simulink subsystem "PvtSubSys_VSM_ALL"  (R2020b)
settings: Solver=VariableStepAuto  StartTime=0.0  StopTime=10.0  RelTol=1e-3
values from neighbouring files (symbols this model uses):
  P_VSM_NOH_Act_Req = 0    [VSM_All.sldd]
  P_VSM_NOH_Swt_Req = 0    [VSM_All.sldd]
undefined symbols (not defined in the file or in its folder): ACC_STATE, HWA_STATE, LCK_STATE, P_VSM_ACCSOS_SW, P_VSM_AESSwtReq, P_VSM_CruiseFunUserInputMappingWays, P_VSM_ELKSwtReq, P_VSM_ESS_VehSwtReq, P_VSM_HWA_DMS_Enable, P_VSM_ICA_HandsOffSwtReq, P_VSM_IntelligentEvaSwtReq, P_VSM_ISLSwtReq, P_VSM_LCKSwtReq, P_VSM_LDWSwtReq, P_VSM_LKASwtReq, P_VSM_LSSSwtReq, P_VSM_PowerTrainConfig, P_VSM_SOSContinueTime, P_VSM_SOSSpdLimit, P_VSM_TSR_Dis_keep_SPL_Table, P_VSM_TSR_Dis_keep_SPLend, P_VSM_TSR_Dis_keep_TS_Table, P_VSM_TSR_Ena_SPLSupp_Table, P_VSM_TSR_Ena_TS_Table, P_VSM_TSR_SLIF_Speed_High, P_VSM_TSR_SLIF_Speed_Low, P_VSM_TSR_SLW_SnvtySwitch, P_VSM_TSR_SLW_Speed_Delta_disable, P_VSM_TSR_SLW_Speed_Delta_enable, P_VSM_TSR_SLW_Speed_High, P_VSM_TSR_SLW_Speed_Low, P_VSM_TSR_SLW_TrafEyeAvtiveDist, P_VSM_TSR_SLW_Warning_Time, P_VSM_TSR_SteerWheelAngle, P_VSM_TSR_SWS_speed_withDir, P_VSM_TSR_SWS_speed_woDir, P_VSM_TSRSwtReq, P_VSM_TSRWarnSwtReq, TJA_STATE, User_LC_ALCswt, User_LC_DrvConfirm, User_LC_DrvLCswt, User_LC_DrvOverride, User_LC_LeTurnNextLineReq, User_LC_RiTurnNextLineReq, User_LC_TurnMostLeLineReq, User_LC_TurnMostRiLineReq, User_LeTurnLmpOn, User_RiTurnLmpOn
libraries: simulink x51
(part 6 of 7)

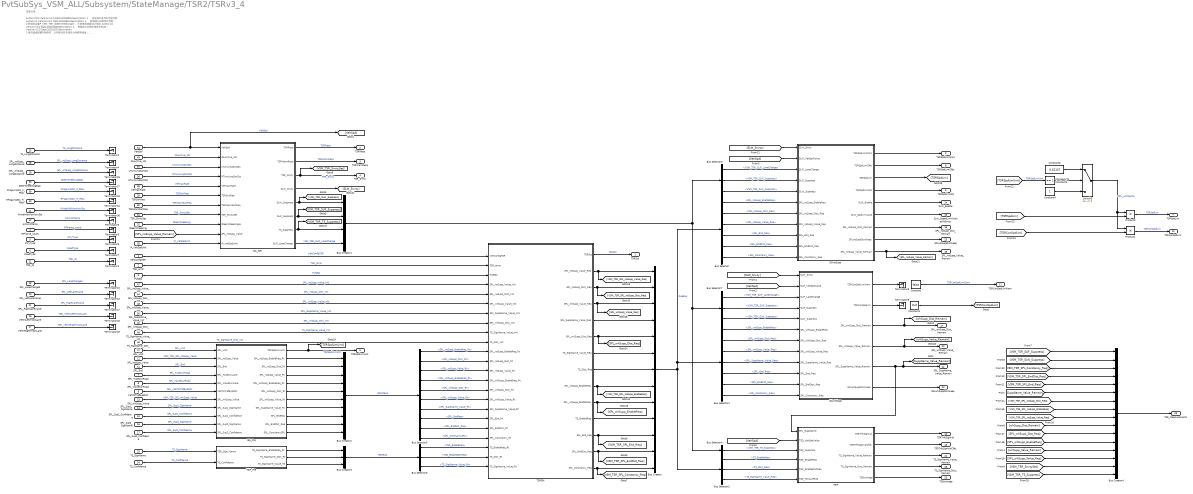
== system PvtSubSys_VSM_ALL/Subsystem/StateManage/TSR2/TSRv3_4 ==
  note: 变更记录
  note: Author:CZN
      | Version:V3.0
      | Data:20200919
      | Description:
      | 1.实现海外版TSR全部功能
      | Author:LC
      | Version:V3.1
      | Data:20200919
      | Description:
      | 1.新增掉头抑制条件判断；
      | 2.新增标定量P_VSM_TSR_SteerWheelAngle；
      | 3.新增观测量CAN输出
      | Author:LC
      | Version:V3.2
      | Data:20201008
      | Description:
      | 1.修复掉头抑制车速条件BUG；
      | Version:V3.3
      | Data:20201102
      | Description:
      | 1.修改超速报警抑制条件，从判断当前车速改为判断限速值；
      | 2.修改TSR_error条件下的状态跳转
      | 3.增加了灵敏度设置限幅；
      | 4.更改SLW_Enable信号来源；
      | 5.修复车速单位为英里时，报警值为公里数值问题；
      | 6.更改限速报警限速策略,改为融合发出信息就显示；
      | Version:V3.4
      | Data:20201103
      | Description:
      | 1、新增三个观测量；
      | 2、新增限速使能触发判断；
      | Version:V3.5
      | Data:20201105
      | Description:
      | 1、按照《交通标志信息功能规范》，新增仪表双位灯输出策略；
      | Version:V3.6
      | Data:20201201
      | Description:
      | 1、条件限速使能改为触发式；
  VehConfigTSR : Inport  OutDataTypeStr=uint8
  TSR_error : Inport  Port=2  OutDataTypeStr=uint8
  FUSSts : Inport  Port=3  OutDataTypeStr=uint8
  RFframe_count : Inport  Port=4  OutDataTypeStr=uint32
  CtryType : Inport  Port=5  OutDataTypeStr=uint8
  RoadType : Inport  Port=6  OutDataTypeStr=uint8
  SPL_TypeCurRoad : Inport  Port=7  OutDataTypeStr=uint8
  SPL_ValueCurRoad : Inport  Port=8  OutDataTypeStr=uint8
  VehToTrafEyeDist : Inport  Port=9  OutDataTypeStr=uint16
  SPL_Unit : Inport  Port=10  OutDataTypeStr=uint8
  SPL_End : Inport  Port=11  OutDataTypeStr=uint8
  SPL_noSupp_Value : Inport  Port=12  OutDataTypeStr=uint8
  SPL_whSupp_Value : Inport  Port=13  OutDataTypeStr=uint8
  SPL_Sup1_SignName : Inport  Port=14  OutDataTypeStr=uint8
  SPL_Sup1_Confidence : Inport  Port=15  OutDataTypeStr=single
  SPL_Sup2_SignName : Inport  Port=16  OutDataTypeStr=uint8
  SPL_Sup2_Confidence : Inport  Port=17  OutDataTypeStr=single
  SPL_noSupp_LongDistance : Inport  Port=18  OutDataTypeStr=uint8
  SPL_whSupp_LongDistance : Inport  Port=19  OutDataTypeStr=uint8
  SPL_LeftLaneValue : Inport  Port=20  OutDataTypeStr=uint8
  SPL_RightLaneValue : Inport  Port=21  OutDataTypeStr=uint8
  TSR_ID : Inport  Port=22  OutDataTypeStr=uint8
  TS_SignName : Inport  Port=23  OutDataTypeStr=uint8
  TS_Confidence : Inport  Port=24  OutDataTypeStr=single
  TS_LongDistance : Inport  Port=25  OutDataTypeStr=uint8
  VehInLeftmostLane : Inport  Port=26  OutDataTypeStr=uint8
  VehInRightmostLane : Inport  Port=27  OutDataTypeStr=uint8
  SPL_LaneChanged : Inport  Port=28  OutDataTypeStr=uint8
  TSRSwtReq : Inport  Port=29  OutDataTypeStr=boolean
  TSRWarnSwtReq : Inport  Port=30  OutDataTypeStr=boolean
  TSR_SnvtySet : Inport  Port=31  OutDataTypeStr=int8
  SteerWheelAng : Inport  Port=32  OutDataTypeStr=single
  SteerWheelAngSign : Inport  Port=33  OutDataTypeStr=boolean
  VehSpd : Inport  Port=34  OutDataTypeStr=single
  IP_VehSpdUnit : Inport  Port=35  OutDataTypeStr=boolean
  RTurnLmpSwtSts : Inport  Port=36  OutDataTypeStr=boolean
  LTurnLmpSwtSts : Inport  Port=37  OutDataTypeStr=boolean
  VehYawRate : Inport  Port=38  OutDataTypeStr=single
  FFogLmpSts_F_Pbox : Inport  Port=39  OutDataTypeStr=boolean
  RFogLmpSts_R_Pbox : Inport  Port=40  OutDataTypeStr=boolean
  WindshldWiprActvSts : Inport  Port=41  OutDataTypeStr=boolean
  ACAmbTemp : Inport  Port=42  OutDataTypeStr=single
  ISLActive_sts : Inport  Port=43  OutDataTypeStr=boolean
  SPL_noSupp_Dist_Init : Inport  Port=44  OutDataTypeStr=single
  SPL_whSupp_Dist_Init : Inport  Port=45  OutDataTypeStr=single
  TS_SignName_Dist_Init : Inport  Port=46  OutDataTypeStr=single
  SPL_noSupp_Value_Init : Inport  Port=47  OutDataTypeStr=uint8
  SPL_whSupp_Value_Init : Inport  Port=48  OutDataTypeStr=uint8
  TS_SignName_Value_Init : Inport  Port=49  OutDataTypeStr=uint8
  SPL_SuppName_Value_Init : Inport  Port=50  OutDataTypeStr=uint8
  Bus Creator : BusCreator  Inputs=13
  Bus Creator1 : BusCreator  Inputs=4
  Bus Creator2 : BusCreator  Inputs=10
  Bus Creator3 : BusCreator  Inputs=3
  Bus Creator4 : BusCreator  Inputs=16
  Bus Selector : BusSelector  OutputSignals=SPL_noSupp_EnableReq,SPL_noSupp_Dist_Req,SPL_noSupp_Value_Req,SPL_End_Req,SPL_EndDist_Req,SPL_Constancy_Req
  Bus Selector1 : BusSelector  OutputSignals=SPL_whSupp_EnableReq,SPL_whSupp_Dist_Req,SPL_whSupp_Value_Req,SPL_SuppName_Value_Req,SPL_End_Req,SPL_EndDist_Req,SPL_Constancy_Req
  Bus Selector2 : BusSelector  OutputSignals=TS_EnableReq,TS_Dist_Req,TS_SignName_Value_Req
  Bus Selector3 : BusSelector  OutputSignals=VSM_TSR_SLIF_LaneChange,VSM_TSR_SLIF_Suppress,VSM_TSR_SLW_Suppress
  Bus Selector4 : BusSelector  OutputSignals=VSM_TSR_TS_Suppress
  Bus Selector5 : BusSelector  OutputSignals=SPL_noSupp_EnableReq_Rt,SPL_noSupp_Dist_Rt,SPL_noSupp_Value_Rt,SPL_whSupp_EnableReq_Rt,SPL_whSupp_Dist_Rt,SPL_whSupp_Value_Rt,SPL_SuppName_Value_Rt,SPL_EndReq,SPL_EndDist_Req,SPL_ConstancySPL
  Bus Selector6 : BusSelector  OutputSignals=TSD_EnableReq,TSD_EnableDistReq,TS_SignName_Value_Rt
  Bus Selector7 : BusSelector  OutputSignals=VSM_TSR_SLIF_LaneChange,VSM_TSR_SLIF_Suppress,VSM_TSR_SLW_Suppress
  Compare To Constant4 : simulink/Logic and Bit Operations/Compare To Constant  relop===  const=1  OutDataTypeStr=boolean
  Constant : Constant  Value=false  OutDataTypeStr=boolean
  Constant1 : Constant  Value=0x0  OutDataTypeStr=uint8
  Constant3 : Constant  Value=0.62137
  Constant4 : Constant
  ISA_Pre : Subsystem
  ISA_Set : Subsystem
  ISAnoSupp : Subsystem
  ISAwhSupp : Subsystem
  Product1 : Product  OutDataTypeStr=uint8
  Product3 : Product  OutDataTypeStr=uint8
  Switch5 : Switch  Criteria=u2 ~= 0  Threshold=1  OutDataTypeStr=single
  TSIF : Subsystem
  TSIF_Pre : Subsystem
  TSRSM : Stateflow chart  TreatAsAtomicUnit=on
  Terminator{1..9,15..19,26..27,33..34,36} (19 alike) : Terminator
  TSRSts : Outport
  TSRResp : Outport  Port=2
  TSRWarnResp : Outport  Port=3
  TSR_Snvty : Outport  Port=4  OutDataTypeStr=int8
  TSRSpdLimUnit : Outport  Port=5
  TSRSpdLimSts : Outport  Port=6  OutDataTypeStr=uint8
  TSRSpdLim : Outport  Port=7  OutDataTypeStr=uint8
  TSRSpdLimCfdc : Outport  Port=8  OutDataTypeStr=uint8
  TSRSpdLimWarn : Outport  Port=9  OutDataTypeStr=boolean
  TSRConSpdLim : Outport  Port=10  OutDataTypeStr=uint8
  TSRConSpdLimWarn : Outport  Port=11  OutDataTypeStr=boolean
  TSRTrfcSignVal : Outport  Port=12  OutDataTypeStr=uint8
  TSRTrfcSignValCfdc : Outport  Port=13  OutDataTypeStr=uint8
  SLW_Enable : Outport  Port=14  OutDataTypeStr=boolean
  SLW_SpeedLimitValueWhSnvty : Outport  Port=15  OutDataTypeStr=uint8
  SPL_noSupp_Dist_Remain : Outport  Port=16  OutDataTypeStr=single
  SPL_whSupp_Dist_Remain : Outport  Port=17
  TS_SignName_Dist_Remain : Outport  Port=18  OutDataTypeStr=single
  SPL_noSupp_Value_Remain : Outport  Port=19  OutDataTypeStr=uint8
  SPL_whSupp_Value_Remain : Outport  Port=20  OutDataTypeStr=uint8
  TS_SignName_Value_Remain : Outport  Port=21  OutDataTypeStr=uint8
  SPL_SuppName_Value_Remain : Outport  Port=22  OutDataTypeStr=uint8
  SPLnoSuppDistKeep : Outport  Port=23  OutDataTypeStr=single
  SPLwhSuppDistKeep : Outport  Port=24  OutDataTypeStr=single
  TSDistKeep : Outport  Port=25
  TSR_Measurements : Outport  Port=26
  wires:
  ISA_Set/2(TSRWarnResp) -> TSRWarnResp/1  "TSRWarnResp"
  SPL_noSupp_LongDistance/1 -> Terminator4/1  "SPL_noSupp_LongDistance"
  FFogLmpSts_F_Pbox/1 -> Terminator33/1  "FFogLmpSts_F_Pbox"
  ISA_Set/8(SLIF_LaneChange) -> Bus Creator1/4  "VSM_TSR_SLIF_LaneChange"
  ISAnoSupp/3(TSRSpdLim) -> [TSRSpdLim]
  FUSSts/1 -> TSRSM/3(FUSSts)  "FUSSts"
  ISAnoSupp/7(SPL_noSupp_Dist_Remain) -> SPL_noSupp_Dist_Remain/1
  VehConfigTSR/1 -> TSRSM/1(VehConfigTSR)  "VehConfigTSR"
  SPL_noSupp_Value/1 -> ISA_Pre/2(SPL_noSupp_Value)  "VSM_TSR_SPL_noSupp_Value"
  Bus Selector/4 -> ISAnoSupp/9(SPL_End_Req)  "<SPL_End_Req>"
  WindshldWiprActvSts/1 -> Terminator36/1  "WindshldWiprActvSts"
  [VehSpd] -> ISAnoSupp/2(SLIF_VehSpdValue)
  RTurnLmpSwtSts/1 -> ISA_Set/4(RTurnLmpSwtSts)  "RTurnLmpSwtSts"
  ISLActive_sts/1 -> ISA_Set/2(ISLActive_sts)  "ISLActive_sts"
  ISAnoSupp/8(SPLnoSuppDistKeep) -> SPLnoSuppDistKeep/1
  Bus Selector/5 -> ISAnoSupp/10(SPL_EndDist_Req)  "<SPL_EndDist_Req>"
  SPL_ValueCurRoad/1 -> ISA_Pre/5(SPL_ValueCurLane)  "SPL_ValueCurRoad"
  ISA_Set/1(TSRResp) -> TSRResp/1  "TSRResp"
  CtryType/1 -> Terminator6/1  "CtryType"
  TSRWarnSwtReq/1 -> ISA_Set/7(TSRWarnSwtReq)  "TSRWarnSwtReq"
  SteerWheelAngSign/1 -> Terminator27/1  "SteerWheelAngSign"
  VehToTrafEyeDist/1 -> ISA_Pre/6(VehToTrafEyeDist)  "SPL_VehToTrafEyeDist"
  ISA_Set/5(SLW_Suppress) -> Bus Creator1/1, [VSM_TSR_SLW_Suppress]
  TS_SignName/1 -> TSIF_Pre/1(TSR_Sign_Name)  "TS_SignName"
  TSRSwtReq/1 -> ISA_Set/6(TSRSwtReq)  "TSRSwtReq"
  TSIF/3(TS_SignName_Value_Remain) -> TS_SignName_Value_Remain/1
  TSIF/1(TSRTrfcSignVal) -> TSRTrfcSignVal/1
  SPL_whSupp_LongDistance/1 -> Terminator26/1  "SPL_whSupp_LongDistance"
  RFframe_count/1 -> Terminator5/1  "RFframe_count"
  SPL_End/1 -> ISA_Pre/3(SPL_End)  "SPL_End"
  TSRSM/1(TSRSts) -> TSRSts/1  "TSRSts"
  ISAwhSupp/5(SPL_SuppName_Value_Remain) -> TSIF/1(SPL_SuppName), [SuppName_Value_Remain], SPL_SuppName_Value_Remain/1
  SPL_LeftLaneValue/1 -> Terminator16/1  "SPL_LeftLaneValue"
  [SLW_Snvty] -> ISAnoSupp/1(SLW_Snvty)
  SteerWheelAng/1 -> ISA_Set/9(SteerWheelAngle)  "SteerWheelAng"
  ISAnoSupp/6(SLW_SpdLimValue) -> SLW_SpeedLimitValueWhSnvty/1
  SPL_LaneChanged/1 -> Terminator15/1  "SPL_LaneChanged"
  VehInRightmostLane/1 -> Terminator19/1  "TSR_VehInRightmostLane"
  SPL_SuppName_Value_Init/1 -> TSRSM/7(SPL_SuppName_Value_Init)  "SPL_SuppName_Value_Init"
  [VehSpd] -> TSIF/2(TSD_VehSpdValue)
  SPL_whSupp_Value/1 -> ISA_Pre/7(SPL_whSupp_Value)  "VSM_TSR_SPL_whSupp_Value"
  RFogLmpSts_R_Pbox/1 -> Terminator34/1  "RFogLmpSts_R_Pbox"
  SPL_whSupp_Value_Init/1 -> TSRSM/6(SPL_whSupp_Value_Init)  "SPL_whSupp_Value_Init"
  ISAnoSupp/4(TSRSpdLimSts) -> TSRSpdLimSts/1
  SPL_noSupp_Dist_Init/1 -> TSRSM/5(SPL_noSupp_Dist_Init)  "SPL_noSupp_Dist_Init"
  LTurnLmpSwtSts/1 -> ISA_Set/3(LTurnLmpSwtSts)  "LTurnLmpSwtSts"
  VehYawRate/1 -> ISA_Set/5(VehYawRate)  "VehYawRate"
  SPL_whSupp_Dist_Init/1 -> TSRSM/8(SPL_whSupp_Dist_Init)  "SPL_whSupp_Dist_Init"
  VehInLeftmostLane/1 -> Terminator18/1  "TSR_VehInLeftmostLane"
  TSR_error/1 -> TSRSM/2(TSR_error)  "TSR_error"
  Bus Selector/6 -> ISAnoSupp/11(SPL_Constancy_Req)  "<SPL_Constancy_Req>"
  TSIF/2(TSRTrfcSignValCfdc) -> TSRTrfcSignValCfdc/1
  TS_SignName_Dist_Init/1 -> TSRSM/10(TS_Dist_Init)  "TS_SignName_Dist_Init"
  Bus Selector3/1 -> ISAnoSupp/3(SLIF_LaneChange)  "<VSM_TSR_SLIF_LaneChange>"
  TS_SignName_Value_Init/1 -> TSRSM/9(TS_SignName_Value_Init)  "TS_SignName_Value_Init"
  SPL_RightLaneValue/1 -> Terminator17/1  "SPL_RightLaneValue"
  TS_LongDistance/1 -> Terminator2/1  "TS_LongDistance"
  ISA_Set/6(SLIF_Suppress) -> Bus Creator1/2, [VSM_TSR_SLIF_Suppress]
  ISAwhSupp/4(SPL_whSupp_Value_Remain) -> [whSupp_Value_Remain], SPL_whSupp_Value_Remain/1
  TSIF/4(TS_SignName_Dist_Remain) -> TS_SignName_Dist_Remain/1
  SPL_TypeCurRoad/1 -> ISA_Pre/4(SPL_TypeCurLane)  "SPL_TypeCurRoad"
  SPL_noSupp_Value_Init/1 -> TSRSM/4(SPL_noSupp_Value_Init)  "SPL_noSupp_Value_Init"
  VehSpd/1 -> [VehSpd], ISA_Set/1(VehSpd)  "VehSpd"
  ISAwhSupp/3(SPL_whSupp_Dist_Remain) -> [whSupp_Dist_Remain], SPL_whSupp_Dist_Remain/1
  ACAmbTemp/1 -> Terminator3/1  "ACAmbTemp"
  RoadType/1 -> Terminator7/1  "RoadType"
  TS_Confidence/1 -> TSIF_Pre/2(TS_Confidence)  "TS_Confidence"
  TSR_ID/1 -> Terminator1/1  "TSR_ID"
  ISAwhSupp/1(TSRConSpdLimWarn) -> Terminator8/1
  ISAwhSupp/2(TSRConSpdLim) -> Terminator9/1
  TSIF_Pre/1(TS_SignName_EnableReq_Rt) -> Bus Creator3/1
  TSIF_Pre/2(TS_SignName_Dist_Rt) -> Bus Creator3/2
  TSIF_Pre/3(TS_SignName_Value_Rt) -> Bus Creator3/3
  SPL_Sup1_SignName/1 -> ISA_Pre/8(SPL_Sup1_SignName)  "SPL_Sup1_SignName"
  SPL_Sup1_Confidence/1 -> ISA_Pre/9(SPL_Sup1_Confidence)  "SPL_Sup1_Confidence"
  SPL_Sup2_SignName/1 -> ISA_Pre/10(SPL_Sup2_SignName)  "SPL_Sup2_SignName"
  SPL_Sup2_Confidence/1 -> ISA_Pre/11(SPL_Sup2_Confidence)  "SPL_Sup2_Confidence"
  ISA_Set/7(TS_Suppress) -> Bus Creator1/3, [VSM_TSR_TS_Suppress]
  Bus Selector2/2 -> TSIF/5(TSIF_EnableDistReq)  "<TS_Dist_Req>"
  Bus Selector2/1 -> TSIF/4(TSIF_EnableReq)  "<TS_EnableReq>"
  Bus Selector4/1 -> TSIF/3(TSIF_Suppress)  "<VSM_TSR_TS_Suppress>"
  ISAnoSupp/5(SLW_Enable) -> SLW_Enable/1
  TSRSM/3(SPL_noSupp_Dist_Req) -> [VSM_TSR_SPL_noSupp_Dist_Req], Bus Creator/2
  TSRSM/2(SPL_noSupp_Value_Req) -> [VSM_TSR_SPL_noSupp_Value_Req], Bus Creator/1
  TSRSM/4(SPL_whSupp_Value_Req) -> [SPL_whSupp_Value_Req], Bus Creator/3
  TSRSM/5(SPL_SuppName_Value_Req) -> Bus Creator/4
  TSRSM/6(SPL_whSupp_Dist_Req) -> [SPL_whSupp_Dist_Req], Bus Creator/5
  TSRSM/7(TS_SignName_Value_Req) -> Bus Creator/6
  TSRSM/8(TS_Dist_Req) -> Bus Creator/7
  TSRSM/9(SPL_noSupp_EnableReq) -> [VSM_TSR_SPL_noSupp_EnableReq], Bus Creator/8
  TSRSM/10(SPL_whSupp_EnableReq) -> [SPL_whSupp_EnableReq], Bus Creator/9
  TSRSM/11(TS_EnableReq) -> Bus Creator/10
  Bus Creator/1 -> Bus Selector2/1, Bus Selector/1, Bus Selector1/1  "ReqBus"
  Bus Selector/1 -> ISAnoSupp/6(SPL_noSupp_EnableReq)  "<SPL_noSupp_EnableReq>"
  Bus Selector2/3 -> TSIF/6(TSD_TSValueReq)  "<TS_SignName_Value_Req>"
  Bus Creator1/1 -> Bus Selector7/1, Bus Selector4/1, Bus Selector3/1
  Bus Selector3/2 -> ISAnoSupp/4(SLIF_Suppress)  "<VSM_TSR_SLIF_Suppress>"
  Bus Selector3/3 -> ISAnoSupp/5(SLW_Suppress)  "<VSM_TSR_SLW_Suppress>"
  ISAnoSupp/1(TSRSpdLimWarn) -> TSRSpdLimWarn/1
  Bus Creator2/1 -> Bus Selector5/1  "SPLRtBus"
  ISA_Pre/2(SPL_noSupp_EnableReq_Rt) -> Bus Creator2/1
  ISA_Pre/3(SPL_noSupp_Dist_Rt) -> Bus Creator2/2
  ISA_Pre/4(SPL_noSupp_Value_Rt) -> Bus Creator2/3
  ISA_Pre/5(SPL_whSupp_EnableReq_Rt) -> Bus Creator2/4
  ISA_Pre/6(SPL_whSupp_Dist_Rt) -> Bus Creator2/5
  ISA_Pre/7(SPL_whSupp_Value_Rt) -> Bus Creator2/6
  ISA_Pre/8(SPL_SuppName_Value_Rt) -> Bus Creator2/7
  ISA_Pre/9(SPL_EndReq) -> Bus Creator2/8
  ISA_Pre/10(SPL_EndDist_Req) -> Bus Creator2/9
  ISA_Pre/11(SPL_ConstancySPL) -> Bus Creator2/10
  Bus Selector5/2 -> TSRSM/12(SPL_noSupp_Dist_Rt)  "<SPL_noSupp_Dist_Rt>"
  Bus Selector5/1 -> TSRSM/11(SPL_noSupp_EnableReq_Rt)  "<SPL_noSupp_EnableReq_Rt>"
  Bus Selector5/3 -> TSRSM/13(SPL_noSupp_Value_Rt)  "<SPL_noSupp_Value_Rt>"
  Bus Selector5/4 -> TSRSM/14(SPL_whSupp_EnableReq_Rt)  "<SPL_whSupp_EnableReq_Rt>"
  Bus Selector5/5 -> TSRSM/15(SPL_whSupp_Dist_Rt)  "<SPL_whSupp_Dist_Rt>"
  Bus Selector5/6 -> TSRSM/16(SPL_whSupp_Value_Rt)  "<SPL_whSupp_Value_Rt>"
  Bus Selector5/7 -> TSRSM/17(SPL_SuppName_Value_Rt)  "<SPL_SuppName_Value_Rt>"
  Bus Creator3/1 -> Bus Selector6/1  "TSRtBus"
  Bus Selector6/1 -> TSRSM/21(TS_EnableReq_Rt)  "<TSD_EnableReq>"
  Bus Selector6/2 -> TSRSM/22(TS_Dist_Rt)  "<TSD_EnableDistReq>"
  Bus Selector6/3 -> TSRSM/23(TS_SignName_Value_Rt)  "<TS_SignName_Value_Rt>"
  Bus Selector5/8 -> TSRSM/18(SPL_End_Rt)  "<SPL_EndReq>"
  Bus Selector5/9 -> TSRSM/19(SPL_EndDist_Rt)  "<SPL_EndDist_Req>"
  TSRSM/12(SPL_End_Req) -> [VSM_TSR_SPL_End_Req], Bus Creator/11
  TSRSM/13(SPL_EndDist_Req) -> [VSM_TSR_SPL_EndDist_Req], Bus Creator/12
  TSRSM/14(SPL_Constancy_Req) -> [VSM_TSR_SPL_Constancy_Req], Bus Creator/13
  SPL_Unit/1 -> ISA_Pre/1(SPL_Unit)  "SPL_Unit"
  TSR_SnvtySet/1 -> ISA_Set/8(TSR_SnvtySet)  "TSR_SnvtySet"
  IP_VehSpdUnit/1 -> ISA_Set/11(IP_VehSpdUnit)  "IP_VehSpdUnit"
  ISA_Pre/1(TSRSpdLimUnit) -> [TSRSpdLimUnit], TSRSpdLimUnit/1  "TSRSpdLimUnit"
  ISA_Set/3(TSR_Snvty) -> TSR_Snvty/1, [VSM_TSR_SnvtySet]  "TSR_Snvty"
  ISA_Set/4(SLW_Snvty) -> [SLW_Snvty]
  Bus Selector1/1 -> ISAwhSupp/6(SPL_whSupp_EnableReq)  "<SPL_whSupp_EnableReq>"
  Bus Selector1/2 -> ISAwhSupp/7(SPL_whSupp_Dist_Req)  "<SPL_whSupp_Dist_Req>"
  Bus Selector1/3 -> ISAwhSupp/8(SPL_whSupp_Value_Req)  "<SPL_whSupp_Value_Req>"
  Bus Selector1/4 -> ISAwhSupp/9(SPL_SuppName_Value_Req)  "<SPL_SuppName_Value_Req>"
  Bus Selector7/3 -> ISAwhSupp/5(SLW_Suppress)  "<VSM_TSR_SLW_Suppress>"
  Bus Selector7/2 -> ISAwhSupp/4(SLIF_Suppress)  "<VSM_TSR_SLIF_Suppress>"
  Bus Selector7/1 -> ISAwhSupp/3(SLIF_LaneChange)  "<VSM_TSR_SLIF_LaneChange>"
  [SLW_Snvty] -> ISAwhSupp/1(SLW_Snvty)
  [VehSpd] -> ISAwhSupp/2(SLIF_VehSpdValue)
  Bus Selector/2 -> ISAnoSupp/7(SPL_noSupp_Dist_Req)  "<SPL_noSupp_Dist_Req>"
  Bus Selector/3 -> ISAnoSupp/8(SPL_noSupp_Value_Req)  "<SPL_noSupp_Value_Req>"
  Bus Selector5/10 -> TSRSM/20(SPL_Constancy_Rt)  "<SPL_ConstancySPL>"
  ISAwhSupp/6(SPLwhSuppDistKeep) -> SPLwhSuppDistKeep/1
  TSIF/5(TSDistKeep) -> TSDistKeep/1
  Bus Creator4/1 -> TSR_Measurements/1
  [VSM_TSR_SPL_noSupp_Dist_Req] -> Bus Creator4/7
  [VSM_TSR_SPL_noSupp_EnableReq] -> Bus Creator4/8
  [SuppName_Value_Remain] -> Bus Creator4/6
  [VSM_TSR_SPL_noSupp_Value_Req] -> Bus Creator4/9
  [VSM_TSR_SPL_EndDist_Req] -> Bus Creator4/4
  [VSM_TSR_SPL_End_Req] -> Bus Creator4/5
  [VSM_TSR_SPL_Constancy_Req] -> Bus Creator4/3
  [VSM_TSR_SLW_Suppress] -> Bus Creator4/2
  [VSM_TSR_SLIF_Suppress] -> Bus Creator4/1
  [whSupp_Dist_Remain] -> Bus Creator4/10
  [SPL_whSupp_Dist_Req] -> Bus Creator4/11
  [SPL_whSupp_EnableReq] -> Bus Creator4/12
  [whSupp_Value_Remain] -> Bus Creator4/13
  [SPL_whSupp_Value_Req] -> Bus Creator4/14
  [VSM_TSR_SnvtySet] -> Bus Creator4/15
  [VSM_TSR_TS_Suppress] -> Bus Creator4/16
  ISAnoSupp/2(TSRSpdLimCfdc) -> TSRSpdLimCfdc/1
  [SPL_noSupp_Value_Remain] -> ISA_Set/10(SPL_noSupp_Value)
  ISAnoSupp/9(SPL_noSupp_Value_Remain) -> SPL_noSupp_Value_Remain/1, [SPL_noSupp_Value_Remain]
  Constant4/1 -> Switch5/3
  Constant3/1 -> Switch5/1
  [TSRSpdLimUnit] -> Compare To Constant4/1  "TSRSpdLimUnit"
  Compare To Constant4/1 -> Switch5/2
  Switch5/1 -> Product1/1, Product3/1  "SPL_unitFactor"
  [TSRSpdLim] -> Product3/2
  Product3/1 -> TSRSpdLim/1  "TSRSpdLim"
  [TSRConSpdLim] -> Product1/2
  Product1/1 -> TSRConSpdLim/1  "TSRConSpdLim"
  Bus Selector1/5 -> ISAwhSupp/10(SPL_End_Req)  "<SPL_End_Req>"
  Bus Selector1/6 -> ISAwhSupp/11(SPL_EndDist_Req)  "<SPL_EndDist_Req>"
  Bus Selector1/7 -> ISAwhSupp/12(SPL_Constancy_Req)  "<SPL_Constancy_Req>"
  Constant/1 -> TSRConSpdLimWarn/1  "TSRConSpdLimWarn"
  Constant1/1 -> [TSRConSpdLim]

== system PvtSubSys_VSM_ALL/Subsystem/StateManage/UOM/GW_V71 ==
  AD : Inport
  FunFeedback : Inport  Port=2
  Bus Selector : BusSelector  OutputSignals=CC_ACC_CRUISE_OFFSwt,CC_ACC_DecSetSpd_SetSwt,CC_ACC_IncSetSpd_ResuSwt,ACC_TimeGap_DecSetSwt,ACC_TimeGap_IncSetSwt,CC_ACC_CANCEL_OFFSwt,CC_ACCSwtErr,HWA_OK_OFFSwt,Start_StopSts,EngState,RTurnLmpSwtSts,LTurnLmpSwtSts,ALC_SwtReq,HWA_SwtReq,HWA_SnvtySet,NOH_Act_Req,NOH_Swt_Req,HCU_PowertrainSts
  Bus Selector1 : BusSelector  OutputSignals=LC_ReqUserConfirm,ISL_ReqUserConfirm
  Bus Creator : BusCreator  Inputs=28
  UOM : Subsystem  ReferencedSubsystem=PvtSubSys_VSM_UOM
      settings: PortSchema="{\"entries\":[{\"content\":{\"sides\":[{\"content\":{\"connectorIds\":[\"In1\",\"In2\",\"In3\",\"In4\",\"In5\",\"In6\",\"In7\",\"In8\",\"In9\",\"In10\",\"In12\",\"In13\",\"In14\",\"In15\",\"In19\",\"In16\",\"In17\",\"In18\",\"In20\",\"In11\"]},\"type\":\"ConnectorPlacement.EquallySpacedRectSide\",\"uuid\":\"8a031895-c628-456d-a98d-aefceead3803\"},{\"content\":{\"connectorIds\":[\"Out1\",\"Out2\",\"Out3\",\"Out4\",\"Out5\",\"Out6\",\"Out7\",\"Out8\",\"Out9\",\"Out10\",\"Out11\",\"Out12\",\"Out13\",\"Out14\",\"Out15\",\"Out16\",\"Out17\",\"Out18\",\"Out19\",\"Out20\",\"Out21\",\"Out22\",\"Out23\",\"Out24\",\"Out25\",\"Out26\",\"Out27\",\"Out28\"],\"side\":\"RIGHT\"},\"type\":\"ConnectorPlacement.EquallySpacedRectSide\",\"uuid\":\"201138b0-f4fb-49c8-a747-ccd5c71c9227\"},{\"content\":{\"connectorIds\":[],\"side\":\"TOP\"},\"type\":\"ConnectorPlacement.EquallySpacedRectSide\",\"uuid\":\"49912179-053f-44be-a038-33ec636c9c18\"},{\"content\":{\"connectorIds\":[],\"side\":\"HIDDEN\"},\"type\":\"ConnectorPlacement.EquallySpacedRectSide\",\"uuid\":\"18e5eac0-8321-4657-a140-4af4811aa693\"}]},\"type\":\"ConnectorPlacement.EquallySpacedConnector\",\"uuid\":\"1536c368-f3b9-40d0-8629-16ae14280190\"}],\"packageUris\":[\"http://schema.mathworks.com/mf0/Connector/R2020b\"],\"version\":\"1.0\"}"
  UserOperation : Outport
  wires:
  Bus Selector/18 -> UOM/18  "<HCU_PowertrainSts>"
  UOM/28 -> Bus Creator/28
  Bus Selector/17 -> UOM/17  "<NOH_Swt_Req>"
  Bus Selector/16 -> UOM/16  "<NOH_Act_Req>"
  UOM/25 -> Bus Creator/25
  UOM/24 -> Bus Creator/24
  UOM/23 -> Bus Creator/23
  Bus Selector/15 -> UOM/19  "<HWA_SnvtySet>"
  FunFeedback/1 -> Bus Selector1/1
  AD/1 -> Bus Selector/1
  Bus Creator/1 -> UserOperation/1
  UOM/13 -> Bus Creator/13
  UOM/14 -> Bus Creator/14
  UOM/7 -> Bus Creator/7
  UOM/8 -> Bus Creator/8
  UOM/10 -> Bus Creator/10
  UOM/5 -> Bus Creator/5
  UOM/4 -> Bus Creator/4
  UOM/2 -> Bus Creator/2
  UOM/1 -> Bus Creator/1
  Bus Selector/2 -> UOM/2  "<CC_ACC_DecSetSpd_SetSwt>"
  UOM/11 -> Bus Creator/11
  UOM/9 -> Bus Creator/9
  Bus Selector/1 -> UOM/1  "<CC_ACC_CRUISE_OFFSwt>"
  Bus Selector/5 -> UOM/5  "<ACC_TimeGap_IncSetSwt>"
  UOM/3 -> Bus Creator/3
  Bus Selector/6 -> UOM/6  "<CC_ACC_CANCEL_OFFSwt>"
  Bus Selector/3 -> UOM/3  "<CC_ACC_IncSetSpd_ResuSwt>"
  Bus Selector/8 -> UOM/8  "<HWA_OK_OFFSwt>"
  UOM/12 -> Bus Creator/12
  Bus Selector/7 -> UOM/7  "<CC_ACCSwtErr>"
  Bus Selector/4 -> UOM/4  "<ACC_TimeGap_DecSetSwt>"
  Bus Selector/9 -> UOM/9  "<Start_StopSts>"
  Bus Selector/10 -> UOM/10  "<EngState>"
  UOM/6 -> Bus Creator/6
  UOM/18 -> Bus Creator/18
  UOM/21 -> Bus Creator/21
  Bus Selector/12 -> UOM/13  "<LTurnLmpSwtSts>"
  Bus Selector/11 -> UOM/12  "<RTurnLmpSwtSts>"
  UOM/19 -> Bus Creator/19
  UOM/20 -> Bus Creator/20
  UOM/15 -> Bus Creator/15
  UOM/16 -> Bus Creator/16
  UOM/17 -> Bus Creator/17
  Bus Selector1/2 -> UOM/11  "<ISL_ReqUserConfirm>"
  Bus Selector1/1 -> UOM/20  "<LC_ReqUserConfirm>"
  Bus Selector/13 -> UOM/14  "<ALC_SwtReq>"
  UOM/22 -> Bus Creator/22
  Bus Selector/14 -> UOM/15  "<HWA_SwtReq>"
  UOM/26 -> Bus Creator/26
  UOM/27 -> Bus Creator/27

== system PvtSubSys_VSM_ALL/Subsystem/StateManage/Cruise/Cruise/VehSpdCalc ==
  VehicleSpd : Inport
  Constant : Constant  Value=1.3  OutDataTypeStr=single
  Gain1 : Gain  Gain=1.03
  Gain2 : Gain  Gain=0.62137  ParamDataTypeStr=single
  Gain3 : Gain
  Sum : Sum  Inputs=|++
  IP_VehSpd_kmh : Outport  OutDataTypeStr=single
  IP_VehSpd_mph : Outport  Port=2  OutDataTypeStr=single
  ESP_VehSpd_kmh : Outport  Port=3
  wires:
  Gain1/1 -> Sum/1
  Constant/1 -> Sum/2
  Sum/1 -> IP_VehSpd_kmh/1, Gain2/1  "IP_VehSpd_kmh"
  VehicleSpd/1 -> Gain3/1, Gain1/1
  Gain2/1 -> IP_VehSpd_mph/1  "IP_VehSpd_mph"
  Gain3/1 -> ESP_VehSpd_kmh/1  "ESP_VehSpd_kmh"

== system PvtSubSys_VSM_ALL/Subsystem/StateManage/LSS/LCK_LKA_LDW_ELKStateMachine3/ELKState_Machine ==
  LaneARe_SP : Inport
  Lane : Inport  Port=2
  TOS_ELK : Inport  Port=3
  LKAState : Inport  Port=4
  FLWhelDy : Inport  Port=5
  FRWhelDy : Inport  Port=6
  IFC_Failsafe : Inport  Port=7
  canHUTELKError : Inport  Port=8
  ADBUS : Inport  Port=9
  VehConfigELK : Inport  Port=10  OutDataTypeStr=uint8
  Bus Creator : BusCreator  Inputs=8
  Bus Selector : BusSelector  OutputSignals=ESSSts,IFC_SnvtySet,TrqK1,canABSVehicleSpd,canABMVehDynYawRate,canESPVDCActive,canESPPTCActive,canESPBTCActive,canABSABSActive,HandsOffDetd,canSASSteerWheelAngle,canEPS_DriverInputTrqValue,canSASSteerWheelSpd,canABMLateralAcce,LongitudeAcc,canESP_MasterCylindBrakePress,canECMAccrPedlPosnDiagc,canEPS_LKATrqOvlDlvdSts,CURRENT_GEAR,canBCMLeftTurnSWSts,canBCMRightTurnSWSts,HandsOffWarnLevel,HWAActive,canHUTELKSwtReq
  Bus Selector1 : BusSelector  OutputSignals=EVI_VehicleSpd_ms,EVI_Kap
  ELK : Subsystem  ReferencedSubsystem=PvtSubSys_VSM_ELK
      settings: PortSchema="{\"entries\":[{\"content\":{\"sides\":[{\"content\":{\"connectorIds\":[\"In1\",\"In2\",\"In3\",\"In5\",\"In6\",\"In7\",\"In8\",\"In9\",\"In33\",\"In34\",\"In4\",\"In10\",\"In11\",\"In12\",\"In13\",\"In14\",\"In15\",\"In16\",\"In17\",\"In18\",\"In19\",\"In20\",\"In21\",\"In22\",\"In23\",\"In24\",\"In25\",\"In26\",\"In27\",\"In28\",\"In29\",\"In30\",\"In31\",\"In32\"]},\"type\":\"ConnectorPlacement.EquallySpacedRectSide\",\"uuid\":\"ceccd110-8e67-4d1a-a2f8-52d3271645ce\"},{\"content\":{\"connectorIds\":[\"Out1\",\"Out2\",\"Out3\",\"Out4\",\"Out5\",\"Out6\",\"Out7\",\"Out8\",\"Out9\",\"Out10\"],\"side\":\"RIGHT\"},\"type\":\"ConnectorPlacement.EquallySpacedRectSide\",\"uuid\":\"e2e06e4b-d051-4398-b377-d931613ba0e4\"},{\"content\":{\"connectorIds\":[],\"side\":\"TOP\"},\"type\":\"ConnectorPlacement.EquallySpacedRectSide\",\"uuid\":\"b57bf514-c41a-4666-9144-d083656f5f87\"},{\"content\":{\"connectorIds\":[],\"side\":\"HIDDEN\"},\"type\":\"ConnectorPlacement.EquallySpacedRectSide\",\"uuid\":\"c1254c06-62b4-402c-b48e-a5575805cf27\"}]},\"type\":\"ConnectorPlacement.EquallySpacedConnector\",\"uuid\":\"10502b58-4e6e-46e2-a225-d9980936a1bb\"}],\"packageUris\":[\"http://schema.mathworks.com/mf0/Connector/R2020b\"],\"version\":\"1.0\"}"
  ELKstate : Outport
  warn : Outport  Port=2
  ELK_Data : Outport  Port=3
  wires:
  Bus Selector/1 -> ELK/34  "<ESSSts>"
  ELK/1 -> ELKstate/1
  ELK/2 -> warn/1
  Bus Selector/24 -> ELK/31  "<canHUTELKSwtReq>"
  Bus Selector/23 -> ELK/30  "<HWAActive>"
  Bus Selector/22 -> ELK/29  "<HandsOffWarnLevel>"
  Bus Selector/21 -> ELK/28  "<canBCMRightTurnSWSts>"
  Bus Selector/20 -> ELK/27  "<canBCMLeftTurnSWSts>"
  Bus Selector/19 -> ELK/26  "<CURRENT_GEAR>"
  Bus Selector/18 -> ELK/25  "<canEPS_LKATrqOvlDlvdSts>"
  Bus Selector/17 -> ELK/24  "<canECMAccrPedlPosnDiagc>"
  Bus Selector/16 -> ELK/23  "<canESP_MasterCylindBrakePress>"
  Bus Selector/15 -> ELK/22  "<LongitudeAcc>"
  Bus Selector/14 -> ELK/21  "<canABMLateralAcce>"
  Bus Selector/13 -> ELK/20  "<canSASSteerWheelSpd>"
  Bus Selector/12 -> ELK/19  "<canEPS_DriverInputTrqValue>"
  Bus Selector/11 -> ELK/18  "<canSASSteerWheelAngle>"
  Bus Selector/10 -> ELK/17  "<HandsOffDetd>"
  Bus Selector/9 -> ELK/16  "<canABSABSActive>"
  Bus Selector/8 -> ELK/15  "<canESPBTCActive>"
  Bus Selector/7 -> ELK/14  "<canESPPTCActive>"
  Bus Selector/6 -> ELK/13  "<canESPVDCActive>"
  Bus Selector/5 -> ELK/12  "<canABMVehDynYawRate>"
  Bus Selector/4 -> ELK/11  "<canABSVehicleSpd>"
  Bus Selector/3 -> ELK/10  "<TrqK1>"
  Bus Selector/2 -> ELK/4  "<IFC_SnvtySet>"
  ELK/7 -> Bus Creator/5  "ELK_Con_AccPedalRate_ELKExit"
  ELK/8 -> Bus Creator/6  "ELK_Con_BrakePressure_ ELKExit"
  ELK/9 -> Bus Creator/7  "ELK_Con_SteerWheelAngle_ ELKExit"
  ELK/10 -> Bus Creator/8  "ELK_Con_SteerWheelSpd_ ELKExit"
  Bus Creator/1 -> ELK_Data/1
  ADBUS/1 -> Bus Selector/1
  LaneARe_SP/1 -> ELK/1
  LKAState/1 -> ELK/6
  FLWhelDy/1 -> ELK/7
  FRWhelDy/1 -> ELK/8
  IFC_Failsafe/1 -> ELK/9
  canHUTELKError/1 -> ELK/33
  VehConfigELK/1 -> ELK/32
  Lane/1 -> Bus Selector1/1
  Bus Selector1/1 -> ELK/2  "<EVI_VehicleSpd_ms>"
  Bus Selector1/2 -> ELK/3  "<EVI_Kap>"
  TOS_ELK/1 -> ELK/5
  ELK/3 -> Bus Creator/1
  ELK/4 -> Bus Creator/2
  ELK/5 -> Bus Creator/3
  ELK/6 -> Bus Creator/4

== system PvtSubSys_VSM_ALL/Subsystem/StateManage/LSS/LCK_LKA_LDW_ELKStateMachine3/Error ==
  IFC_FailSafe : Inport
  LCKError : Inport  Port=2
  LKAError : Inport  Port=3
  LDWError : Inport  Port=4
  ELKError : Inport  Port=5
  FailSafe : Outport
  LCK_Error : Outport  Port=2
  LKA_Error : Outport  Port=3
  LDW_Error : Outport  Port=4
  ELK_Error : Outport  Port=5
  wires:
  ELKError/1 -> ELK_Error/1
  LDWError/1 -> LDW_Error/1
  LKAError/1 -> LKA_Error/1
  LCKError/1 -> LCK_Error/1
  IFC_FailSafe/1 -> FailSafe/1

== system PvtSubSys_VSM_ALL/Subsystem/StateManage/LSS/LCK_LKA_LDW_ELKStateMachine3/LCK ==
  LCK_Error : Inport  OutDataTypeStr=uint8
  VehConfig : Inport  Port=2
  LKA_LDW_Signal : Inport  Port=3
  ADmix : Inport  Port=4
  LaneARe_SP : Inport  Port=5
  PiloSts : Inport  Port=6
  Lane : Inport  Port=7
  Bus Creator : BusCreator  Inputs=6
  Bus Selector21 : BusSelector  OutputSignals=VehConfigLCK
  Bus Selector22 : BusSelector  OutputSignals=FLWhelDy,FRWhelDy
  Bus Selector23 : BusSelector  OutputSignals=HWAActive,TJAOn,TJASts,canHUTLCKSwtReq,LSSSwtReq,canABSVehicleSpd,canABMVehDynYawRate,canBCMLeftTurnSWSts,canBCMRightTurnSWSts,canECMAccrPedlPosnDiagc,canSASSteerWheelSpd,canESP_MasterCylindBrakePress,canEPS_DriverInputTrqValue,canEPS_LKATrqOvlDlvdSts,TrqK1,canESPVDCActive,canESPPTCActive,canESPBTCActive,canABSABSActive,HandsOffWarnLevel,canSASSteerWheelAngle,canABMLateralAcce,LongitudeAcc,HandsOffDetd,TJALineValid,ESSSts,HWASts,CURRENT_GEAR,LCKLineValid,HWALineValid,BrkPedalSts
  Data Type Conversion : DataTypeConversion  OutDataTypeStr=uint8
  Data Type Conversion1 : DataTypeConversion  OutDataTypeStr=uint8
  LCK : Subsystem  ReferencedSubsystem=PvtSubSys_VSM_LCK
  LCKData : Outport
  LCK_Warn : Outport  Port=2
  LCK_State : Outport  Port=3
  TJA_LCKState : Outport  Port=4
  wires:
  Bus Selector23/31 -> LCK/41  "<BrkPedalSts>"
  Lane/1 -> LCK/37
  PiloSts/1 -> LCK/36
  LaneARe_SP/1 -> LCK/35
  Bus Selector23/30 -> LCK/34  "<HWALineValid>"
  Bus Selector23/29 -> LCK/33  "<LCKLineValid>"
  LCK/9 -> TJA_LCKState/1
  Data Type Conversion/1 -> LCK/31
  Data Type Conversion1/1 -> LCK/7
  Bus Selector23/3 -> Data Type Conversion1/1  "<TJASts>"
  LCK/1 -> LCK_Warn/1  "LCKWarning"
  Bus Selector23/27 -> Data Type Conversion/1  "<HWASts>"
  Bus Creator/1 -> LCKData/1
  LCK/8 -> Bus Creator/6
  LCK/7 -> Bus Creator/5
  LCK/6 -> Bus Creator/4
  LCK/5 -> Bus Creator/3
  LCK/4 -> Bus Creator/2
  Bus Selector21/1 -> LCK/2  "<VehConfigLCK>"
  Bus Selector23/28 -> LCK/32  "<CURRENT_GEAR>"
  Bus Selector23/10 -> LCK/14  "<canECMAccrPedlPosnDiagc>"
  Bus Selector23/6 -> LCK/10  "<canABSVehicleSpd>"
  Bus Selector23/7 -> LCK/11  "<canABMVehDynYawRate>"
  VehConfig/1 -> Bus Selector21/1
  Bus Selector23/18 -> LCK/22  "<canESPBTCActive>"
  Bus Selector23/20 -> LCK/24  "<HandsOffWarnLevel>"
  Bus Selector23/26 -> LCK/30  "<ESSSts>"
  Bus Selector23/16 -> LCK/20  "<canESPVDCActive>"
  Bus Selector23/24 -> LCK/28  "<HandsOffDetd>"
  Bus Selector23/21 -> LCK/25  "<canSASSteerWheelAngle>"
  Bus Selector23/12 -> LCK/16  "<canESP_MasterCylindBrakePress>"
  LCK/3 -> Bus Creator/1
  Bus Selector23/9 -> LCK/13  "<canBCMRightTurnSWSts>"
  Bus Selector23/22 -> LCK/26  "<canABMLateralAcce>"
  Bus Selector23/17 -> LCK/21  "<canESPPTCActive>"
  LCK_Error/1 -> LCK/1
  Bus Selector23/25 -> LCK/29  "<TJALineValid>"
  Bus Selector23/4 -> LCK/8  "<canHUTLCKSwtReq>"
  Bus Selector23/11 -> LCK/15  "<canSASSteerWheelSpd>"
  Bus Selector23/13 -> LCK/17  "<canEPS_DriverInputTrqValue>"
  Bus Selector23/23 -> LCK/27  "<LongitudeAcc>"
  Bus Selector23/8 -> LCK/12  "<canBCMLeftTurnSWSts>"
  Bus Selector23/1 -> LCK/5  "<HWAActive>"
  ADmix/1 -> Bus Selector23/1
  Bus Selector23/15 -> LCK/19  "<TrqK1>"
  Bus Selector23/5 -> LCK/9  "<LSSSwtReq>"
  LCK/2 -> LCK_State/1
  Bus Selector23/14 -> LCK/18  "<canEPS_LKATrqOvlDlvdSts>"
  Bus Selector22/1 -> LCK/3  "<FLWhelDy>"
  Bus Selector23/2 -> LCK/6  "<TJAOn>"
  LKA_LDW_Signal/1 -> Bus Selector22/1
  Bus Selector23/19 -> LCK/23  "<canABSABSActive>"
  Bus Selector22/2 -> LCK/4  "<FRWhelDy>"

== system PvtSubSys_VSM_ALL/Subsystem/StateManage/LSS/LCK_LKA_LDW_ELKStateMachine3/LDW ==
  VehConfig : Inport
  LDW_Error : Inport  Port=2
  LKA_LDW_Signal : Inport  Port=3
  LaneARe_SP : Inport  Port=4
  ADmix : Inport  Port=5
  FailSafe : Inport  Port=6
  ADmix1 : InportShadow  Port=5
  Bus Creator : BusCreator  Inputs=5
  Bus Creator1 : BusCreator  Inputs=4
  Bus Selector14 : BusSelector  OutputSignals=IFC_SnvtySet
  Bus Selector16 : BusSelector  OutputSignals=Scene_LaneValid,HeadingAngle_In,HeadingAngle_Out,LaneCurve,LeftChange,RightChange
  Bus Selector2 : BusSelector  OutputSignals=C_Lanewidth,LeftValid_Valid,RightValid_Valid,Host_LRE,Host_RRE
  Bus Selector3 : BusSelector  OutputSignals=FLWhelDy,FRWhelDy,preFLWhelDy,preFRWhelDy
  Bus Selector5 : BusSelector  OutputSignals=VehConfigLDW
  Bus Selector6 : BusSelector  OutputSignals=LSSSwtReq,canHUTLDWSwtReq,HWAActive,canSASSteerWheelAngle,canEPS_DriverInputTrqValue,canSASSteerWheelSpd,canABMLateralAcce,LongitudeAcc,canESP_MasterCylindBrakePress,canECMAccrPedlPosnDiagc,canEPS_LKATrqOvlDlvdSts,CURRENT_GEAR,canBCMLeftTurnSWSts,canBCMRightTurnSWSts,canABMVehDynYawRate,canESPVDCActive,canESPPTCActive,canESPBTCActive,canABSABSActive,canABSVehicleSpd,ESSSts
  Data Type Conversion : DataTypeConversion  OutDataTypeStr=uint8
  LDW : Subsystem  ReferencedSubsystem=PvtSubSys_VSM_LDW
  LaneARe_SP1 : InportShadow  Port=4
  LaneARe_SP2 : InportShadow  Port=4
  LDW_State : Outport
  LDWData : Outport  Port=2
  LDWCondition : Outport  Port=3
  wires:
  LaneARe_SP2/1 -> LDW/41
  Bus Selector16/3 -> LDW/36  "<HeadingAngle_Out>"
  Data Type Conversion/1 -> LDW/33
  Bus Creator1/1 -> LDWCondition/1
  LDW/10 -> Bus Creator1/4
  LDW/9 -> Bus Creator1/3
  LDW/8 -> Bus Creator1/2
  LDW/7 -> Bus Creator1/1
  Bus Creator/1 -> LDWData/1
  Bus Selector6/16 -> LDW/28  "<canESPVDCActive>"
  Bus Selector6/13 -> LDW/25  "<canBCMLeftTurnSWSts>"
  Bus Selector14/1 -> LDW/1  "<IFC_SnvtySet>"
  Bus Selector6/19 -> LDW/31  "<canABSABSActive>"
  LDW/3 -> Bus Creator/2
  Bus Selector16/5 -> LDW/38  "<LeftChange>"
  Bus Selector6/5 -> LDW/17  "<canEPS_DriverInputTrqValue>"
  Bus Selector6/18 -> LDW/30  "<canESPBTCActive>"
  Bus Selector6/14 -> LDW/26  "<canBCMRightTurnSWSts>"
  Bus Selector2/2 -> LDW/9  "<LeftValid_Valid>"
  LaneARe_SP1/1 -> Bus Selector16/1
  Bus Selector6/2 -> LDW/14  "<canHUTLDWSwtReq>"
  Bus Selector2/5 -> LDW/12  "<Host_RRE>"
  LDW/6 -> Bus Creator/5
  ADmix1/1 -> Bus Selector14/1
  Bus Selector6/15 -> LDW/27  "<canABMVehDynYawRate>"
  Bus Selector3/1 -> LDW/4  "<FLWhelDy>"
  Bus Selector6/8 -> LDW/20  "<LongitudeAcc>"
  Bus Selector2/3 -> LDW/10  "<RightValid_Valid>"
  Bus Selector6/17 -> LDW/29  "<canESPPTCActive>"
  LDW/2 -> Bus Creator/1
  ADmix/1 -> Bus Selector6/1
  LDW_Error/1 -> LDW/3
  Bus Selector2/1 -> LDW/8  "<C_Lanewidth>"
  Bus Selector16/4 -> LDW/37  "<LaneCurve>"
  Bus Selector6/9 -> LDW/21  "<canESP_MasterCylindBrakePress>"
  Bus Selector6/10 -> LDW/22  "<canECMAccrPedlPosnDiagc>"
  LKA_LDW_Signal/1 -> Bus Selector3/1
  FailSafe/1 -> LDW/40
  Bus Selector6/20 -> LDW/32  "<canABSVehicleSpd>"
  Bus Selector2/4 -> LDW/11  "<Host_LRE>"
  LaneARe_SP/1 -> Bus Selector2/1
  Bus Selector6/6 -> LDW/18  "<canSASSteerWheelSpd>"
  Bus Selector5/1 -> LDW/2  "<VehConfigLDW>"
  Bus Selector3/4 -> LDW/7  "<preFRWhelDy>"
  Bus Selector6/1 -> LDW/13  "<LSSSwtReq>"
  Bus Selector3/3 -> LDW/6  "<preFLWhelDy>"
  Bus Selector6/3 -> LDW/15  "<HWAActive>"
  Bus Selector6/12 -> LDW/24  "<CURRENT_GEAR>"
  Bus Selector16/1 -> LDW/34  "<Scene_LaneValid>"
  Bus Selector3/2 -> LDW/5  "<FRWhelDy>"
  Bus Selector16/6 -> LDW/39  "<RightChange>"
  VehConfig/1 -> Bus Selector5/1
  Bus Selector6/7 -> LDW/19  "<canABMLateralAcce>"
  Bus Selector6/4 -> LDW/16  "<canSASSteerWheelAngle>"
  LDW/1 -> LDW_State/1
  Bus Selector6/11 -> LDW/23  "<canEPS_LKATrqOvlDlvdSts>"
  Bus Selector6/21 -> Data Type Conversion/1  "<ESSSts>"
  Bus Selector16/2 -> LDW/35  "<HeadingAngle_In>"
  LDW/4 -> Bus Creator/3
  LDW/5 -> Bus Creator/4

== system PvtSubSys_VSM_ALL/Subsystem/StateManage/LSS/LCK_LKA_LDW_ELKStateMachine3/LKA ==
  LaneARe_SP : Inport
  LKA_LDW_Signal : Inport  Port=2
  LKA_Error : Inport  Port=3  OutDataTypeStr=uint8
  VehConfig : Inport  Port=4
  ADmix : Inport  Port=5
  FailSafe : Inport  Port=6
  ADmix1 : InportShadow  Port=5
  ADmix2 : InportShadow  Port=5
  Bus Creator : BusCreator  Inputs=6
  Bus Creator1 : BusCreator  Inputs=4
  Bus Selector10 : BusSelector  OutputSignals=FLWhelDy,FRWhelDy,preFLWhelDy,preFRWhelDy
  Bus Selector15 : BusSelector  OutputSignals=LSSSwtReq,canHUTLKASwtReq,canHUTELKSwtReq,HWAActive,canABSVehicleSpd,canABMVehDynYawRate,canESPVDCActive,canESPPTCActive,canESPBTCActive,canABSABSActive,TJASts
  Bus Selector17 : BusSelector  OutputSignals=IFC_SnvtySet
  Bus Selector18 : BusSelector  OutputSignals=VehConfigLKA
  Bus Selector19 : BusSelector  OutputSignals=HeadingAngle_In,HeadingAngle_Out,LaneCurve,LeftChange,RightChange,Scene_LaneValid
  Bus Selector20 : BusSelector  OutputSignals=HandsOffDetd,canSASSteerWheelAngle,canEPS_DriverInputTrqValue,canSASSteerWheelSpd,canABMLateralAcce,LongitudeAcc,canESP_MasterCylindBrakePress,canECMAccrPedlPosnDiagc,canEPS_LKATrqOvlDlvdSts,CURRENT_GEAR,canBCMLeftTurnSWSts,canBCMRightTurnSWSts,HandsOffWarnLevel,TrqK1,ESSSts
  Bus Selector7 : BusSelector  OutputSignals=C_Lanewidth,LeftValid_Valid,RightValid_Valid,Host_LRE,Host_RRE,T_A0,T_A1
  Data Type Conversion : DataTypeConversion  OutDataTypeStr=boolean
  Data Type Conversion1 : DataTypeConversion  OutDataTypeStr=uint8
  LKA : Subsystem  ReferencedSubsystem=PvtSubSys_VSM_LKA
  LaneARe_SP1 : InportShadow
  LaneARe_SP2 : InportShadow
  LKAData : Outport
  LKA_State : Outport  Port=2
  LKADesLaneDyoffset_m : Outport  Port=3
  LKA_Warn : Outport  Port=4
  LKA_LKAactive : Outport  Port=5
  LKA_LKAout : Outport  Port=6
  LKA_InterventionEnd : Outport  Port=7
  LKACondition : Outport  Port=8
  wires:
  LaneARe_SP2/1 -> LKA/26
  Bus Selector15/11 -> LKA/25  "<TJASts>"
  Data Type Conversion1/1 -> LKA/48
  Data Type Conversion/1 -> LKA/18
  Bus Creator1/1 -> LKACondition/1
  LKA/16 -> Bus Creator1/4
  LKA/15 -> Bus Creator1/3
  LKA/14 -> Bus Creator1/2
  LKA/13 -> Bus Creator1/1
  Bus Creator/1 -> LKAData/1
  LKA/12 -> Bus Creator/6
  LKA/11 -> Bus Creator/5
  LKA/10 -> Bus Creator/4
  LKA/9 -> Bus Creator/3
  LKA/8 -> Bus Creator/2
  LKA/7 -> Bus Creator/1
  Bus Selector20/9 -> LKA/42  "<canEPS_LKATrqOvlDlvdSts>"
  Bus Selector15/5 -> LKA/19  "<canABSVehicleSpd>"
  ADmix/1 -> Bus Selector15/1
  LKA/2 -> LKADesLaneDyoffset_m/1
  Bus Selector19/4 -> LKA/30  "<LeftChange>"
  Bus Selector7/3 -> LKA/4  "<RightValid_Valid>"
  LKA/1 -> LKA_State/1
  Bus Selector20/3 -> LKA/36  "<canEPS_DriverInputTrqValue>"
  LKA/4 -> LKA_LKAactive/1
  Bus Selector20/14 -> LKA/47  "<TrqK1>"
  Bus Selector19/6 -> LKA/32  "<Scene_LaneValid>"
  Bus Selector20/5 -> LKA/38  "<canABMLateralAcce>"
  Bus Selector19/5 -> LKA/31  "<RightChange>"
  FailSafe/1 -> LKA/33
  LKA/5 -> LKA_LKAout/1
  Bus Selector7/7 -> LKA/8  "<T_A1>"
  LKA_Error/1 -> LKA/13
  Bus Selector20/15 -> Data Type Conversion1/1  "<ESSSts>"
  ADmix2/1 -> Bus Selector17/1
  Bus Selector15/2 -> LKA/16  "<canHUTLKASwtReq>"
  Bus Selector20/7 -> LKA/40  "<canESP_MasterCylindBrakePress>"
  Bus Selector20/4 -> LKA/37  "<canSASSteerWheelSpd>"
  Bus Selector15/8 -> LKA/22  "<canESPPTCActive>"
  LaneARe_SP1/1 -> Bus Selector19/1
  Bus Selector18/1 -> LKA/14  "<VehConfigLKA>"
  Bus Selector20/6 -> LKA/39  "<LongitudeAcc>"
  Bus Selector17/1 -> LKA/1  "<IFC_SnvtySet>"
  LKA/3 -> LKA_Warn/1
  LKA/6 -> LKA_InterventionEnd/1
  Bus Selector20/8 -> LKA/41  "<canECMAccrPedlPosnDiagc>"
  Bus Selector15/3 -> LKA/17  "<canHUTELKSwtReq>"
  Bus Selector19/3 -> LKA/29  "<LaneCurve>"
  LaneARe_SP/1 -> Bus Selector7/1
  Bus Selector15/4 -> Data Type Conversion/1  "<HWAActive>"
  VehConfig/1 -> Bus Selector18/1
  Bus Selector15/6 -> LKA/20  "<canABMVehDynYawRate>"
  Bus Selector20/12 -> LKA/45  "<canBCMRightTurnSWSts>"
  Bus Selector7/1 -> LKA/2  "<C_Lanewidth>"
  Bus Selector20/11 -> LKA/44  "<canBCMLeftTurnSWSts>"
  ADmix1/1 -> Bus Selector20/1
  Bus Selector19/2 -> LKA/28  "<HeadingAngle_Out>"
  Bus Selector15/9 -> LKA/23  "<canESPBTCActive>"
  Bus Selector7/6 -> LKA/7  "<T_A0>"
  Bus Selector10/3 -> LKA/11  "<preFLWhelDy>"
  Bus Selector20/10 -> LKA/43  "<CURRENT_GEAR>"
  Bus Selector7/4 -> LKA/5  "<Host_LRE>"
  Bus Selector10/4 -> LKA/12  "<preFRWhelDy>"
  Bus Selector10/1 -> LKA/9  "<FLWhelDy>"
  Bus Selector20/1 -> LKA/34  "<HandsOffDetd>"
  Bus Selector15/7 -> LKA/21  "<canESPVDCActive>"
  Bus Selector7/2 -> LKA/3  "<LeftValid_Valid>"
  Bus Selector19/1 -> LKA/27  "<HeadingAngle_In>"
  Bus Selector10/2 -> LKA/10  "<FRWhelDy>"
  Bus Selector15/1 -> LKA/15  "<LSSSwtReq>"
  Bus Selector15/10 -> LKA/24  "<canABSABSActive>"
  Bus Selector7/5 -> LKA/6  "<Host_RRE>"
  LKA_LDW_Signal/1 -> Bus Selector10/1
  Bus Selector20/2 -> LKA/35  "<canSASSteerWheelAngle>"
  Bus Selector20/13 -> LKA/46  "<HandsOffWarnLevel>"

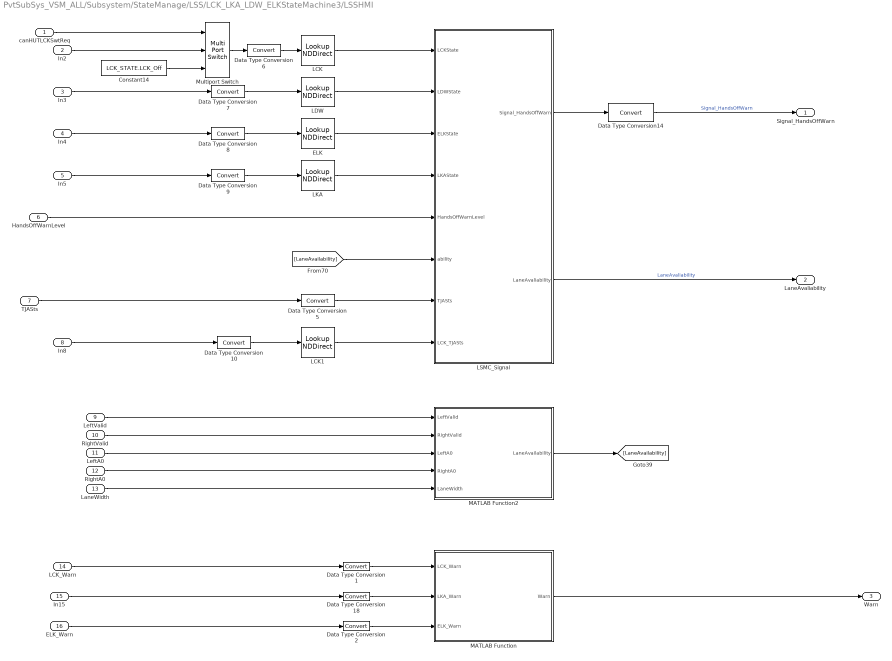
== system PvtSubSys_VSM_ALL/Subsystem/StateManage/LSS/LCK_LKA_LDW_ELKStateMachine3/LSSHMI ==
  canHUTLCKSwtReq : Inport
  In2 : Inport  Port=2
  In3 : Inport  Port=3
  In4 : Inport  Port=4
  In5 : Inport  Port=5
  HandsOffWarnLevel : Inport  Port=6
  TJASts : Inport  Port=7
  In8 : Inport  Port=8
  LeftValid : Inport  Port=9
  RightValid : Inport  Port=10
  LeftA0 : Inport  Port=11
  RightA0 : Inport  Port=12
  LaneWidth : Inport  Port=13
  LCK_Warn : Inport  Port=14
  In15 : Inport  Port=15
  ELK_Warn : Inport  Port=16
  Constant14 : Constant  Value=LCK_STATE.LCK_Off
  Data Type Conversion{1..2,5..10,14,18} (10 alike) : DataTypeConversion
  ELK : LookupNDDirect  NumberOfTableDimensions=1  Table=[0 0 1 1 1 1 1 1 1 0]
  LCK : LookupNDDirect  NumberOfTableDimensions=1  Table=[0 0 1 1 0 0 0 0]
  LCK1 : LookupNDDirect  NumberOfTableDimensions=1  Table=[0 0 1 1 0 0 0 0]
  LDW : LookupNDDirect  NumberOfTableDimensions=1  Table=[0 0 1 0 1 1 0 0]
  LKA : LookupNDDirect  NumberOfTableDimensions=1  Table=[0 0 1 0 1 1 0 0]
  LSMC_Signal : MATLAB Function  TreatAsAtomicUnit=on
  MATLAB Function : MATLAB Function  TreatAsAtomicUnit=on
  MATLAB Function2 : MATLAB Function  TreatAsAtomicUnit=on
  Multiport Switch : MultiPortSwitch  Inputs=2  DiagnosticForDefault=None
  Signal_HandsOffWarn : Outport
  LaneAvaliability : Outport  Port=2
  Warn : Outport  Port=3
  wires:
  Data Type Conversion2/1 -> MATLAB Function/3(ELK_Warn)
  Data Type Conversion1/1 -> MATLAB Function/1(LCK_Warn)
  In15/1 -> Data Type Conversion18/1
  In2/1 -> Multiport Switch/2
  LeftValid/1 -> MATLAB Function2/1(LeftValid)
  TJASts/1 -> Data Type Conversion5/1
  canHUTLCKSwtReq/1 -> Multiport Switch/1
  In8/1 -> Data Type Conversion10/1
  Data Type Conversion14/1 -> Signal_HandsOffWarn/1  "Signal_HandsOffWarn"
  HandsOffWarnLevel/1 -> LSMC_Signal/5(HandsOffWarnLevel)
  MATLAB Function/1(Warn) -> Warn/1
  LCK_Warn/1 -> Data Type Conversion1/1
  In4/1 -> Data Type Conversion8/1
  LeftA0/1 -> MATLAB Function2/3(LeftA0)
  In3/1 -> Data Type Conversion7/1
  LSMC_Signal/2(LaneAvaliability) -> LaneAvaliability/1  "LaneAvaliability"
  In5/1 -> Data Type Conversion9/1
  LSMC_Signal/1(Signal_HandsOffWarn) -> Data Type Conversion14/1
  LKA/1 -> LSMC_Signal/4(LKAState)
  RightA0/1 -> MATLAB Function2/4(RightA0)
  LDW/1 -> LSMC_Signal/2(LDWState)
  LCK1/1 -> LSMC_Signal/8(LCK_TJASts)
  ELK/1 -> LSMC_Signal/3(ELKState)
  Data Type Conversion6/1 -> LCK/1
  Data Type Conversion7/1 -> LDW/1
  LCK/1 -> LSMC_Signal/1(LCKState)
  Constant14/1 -> Multiport Switch/3
  Data Type Conversion10/1 -> LCK1/1
  RightValid/1 -> MATLAB Function2/2(RightValid)
  Data Type Conversion5/1 -> LSMC_Signal/7(TJASts)
  MATLAB Function2/1(LaneAvailability) -> [LaneAvailability]
  Data Type Conversion9/1 -> LKA/1
  [LaneAvailability] -> LSMC_Signal/6(ability)
  Data Type Conversion8/1 -> ELK/1
  Data Type Conversion18/1 -> MATLAB Function/2(LKA_Warn)
  Multiport Switch/1 -> Data Type Conversion6/1
  LaneWidth/1 -> MATLAB Function2/5(LaneWidth)
  ELK_Warn/1 -> Data Type Conversion2/1

== system PvtSubSys_VSM_ALL/Subsystem/StateManage/LSS/TargetLineSelect/ESSLine ==
  In1 : Inport
  In2 : Inport  Port=2
  In3 : Inport  Port=3
  In4 : Inport  Port=4
  In5 : Inport  Port=5
  In6 : Inport  Port=6
  Action Port : ActionPort
  Mux : Mux  Inputs=6
  Out1 : Outport
  wires:
  Mux/1 -> Out1/1
  In1/1 -> Mux/1
  In2/1 -> Mux/2
  In3/1 -> Mux/3
  In6/1 -> Mux/6
  In4/1 -> Mux/4
  In5/1 -> Mux/5

== system PvtSubSys_VSM_ALL/Subsystem/StateManage/LSS/TargetLineSelect/LCKLineS ==
  In1 : Inport
  In2 : Inport  Port=2
  In3 : Inport  Port=3
  In4 : Inport  Port=4
  In5 : Inport  Port=5
  In6 : Inport  Port=6
  Action Port : ActionPort
  Mux : Mux  Inputs=6
  Out1 : Outport
  wires:
  In1/1 -> Mux/1
  In2/1 -> Mux/2
  Mux/1 -> Out1/1
  In3/1 -> Mux/3
  In4/1 -> Mux/4
  In5/1 -> Mux/5
  In6/1 -> Mux/6

== system PvtSubSys_VSM_ALL/Subsystem/StateManage/LSS/TargetLineSelect/LCKLineS1 ==
  In1 : Inport
  In2 : Inport  Port=2
  In3 : Inport  Port=3
  In4 : Inport  Port=4
  In5 : Inport  Port=5
  In6 : Inport  Port=6
  Action Port : ActionPort
  Mux : Mux  Inputs=6
  Out1 : Outport
  wires:
  Mux/1 -> Out1/1
  In4/1 -> Mux/4
  In3/1 -> Mux/3
  In2/1 -> Mux/2
  In5/1 -> Mux/5
  In1/1 -> Mux/1
  In6/1 -> Mux/6

== system PvtSubSys_VSM_ALL/Subsystem/StateManage/LSS/TargetLineSelect/LCKLineS10 ==
  In1 : Inport
  In2 : Inport  Port=2
  In3 : Inport  Port=3
  In4 : Inport  Port=4
  In5 : Inport  Port=5
  In6 : Inport  Port=6
  In7 : Inport  Port=7
  Action Port : ActionPort
  Add1 : Sum
  Mux : Mux  Inputs=6
  Out1 : Outport
  wires:
  In7/1 -> Add1/2
  In5/1 -> Add1/1
  Add1/1 -> Mux/5
  In3/1 -> Mux/3
  In2/1 -> Mux/2
  In4/1 -> Mux/4
  In1/1 -> Mux/1
  In6/1 -> Mux/6
  Mux/1 -> Out1/1

== system PvtSubSys_VSM_ALL/Subsystem/StateManage/LSS/TargetLineSelect/LCKLineS2 ==
  In1 : Inport
  In2 : Inport  Port=2
  In3 : Inport  Port=3
  In4 : Inport  Port=4
  In5 : Inport  Port=5
  In6 : Inport  Port=6
  Action Port : ActionPort
  Mux : Mux  Inputs=6
  Out1 : Outport
  wires:
  In5/1 -> Mux/5
  In4/1 -> Mux/4
  In6/1 -> Mux/6
  In3/1 -> Mux/3
  In2/1 -> Mux/2
  In1/1 -> Mux/1
  Mux/1 -> Out1/1

== system PvtSubSys_VSM_ALL/Subsystem/StateManage/LSS/TargetLineSelect/LCKLineS3 ==
  In1 : Inport
  In2 : Inport  Port=2
  In3 : Inport  Port=3
  In4 : Inport  Port=4
  In5 : Inport  Port=5
  In6 : Inport  Port=6
  Action Port : ActionPort
  In10 : InportShadow  Port=4
  In11 : InportShadow  Port=5
  In12 : InportShadow  Port=6
  In7 : InportShadow
  In8 : InportShadow  Port=2
  In9 : InportShadow  Port=3
  Mux : Mux  Inputs=6
  Mux1 : Mux  Inputs=6
  Out1 : Outport
  Out2 : Outport  Port=2
  wires:
  In12/1 -> Mux1/6
  In11/1 -> Mux1/5
  In10/1 -> Mux1/4
  In9/1 -> Mux1/3
  In8/1 -> Mux1/2
  In7/1 -> Mux1/1
  Mux1/1 -> Out2/1
  Mux/1 -> Out1/1
  In6/1 -> Mux/6
  In4/1 -> Mux/4
  In3/1 -> Mux/3
  In2/1 -> Mux/2
  In1/1 -> Mux/1
  In5/1 -> Mux/5

== system PvtSubSys_VSM_ALL/Subsystem/StateManage/LSS/TargetLineSelect/LCKLineS6 ==
  In1 : Inport
  In2 : Inport  Port=2
  In3 : Inport  Port=3
  In4 : Inport  Port=4
  In5 : Inport  Port=5
  In6 : Inport  Port=6
  Action Port : ActionPort
  In10 : InportShadow  Port=4
  In11 : InportShadow  Port=5
  In12 : InportShadow  Port=6
  In7 : InportShadow
  In8 : InportShadow  Port=2
  In9 : InportShadow  Port=3
  Mux : Mux  Inputs=6
  Mux1 : Mux  Inputs=6
  Out1 : Outport
  Out2 : Outport  Port=2
  wires:
  In5/1 -> Mux/5
  In1/1 -> Mux/1
  In2/1 -> Mux/2
  In3/1 -> Mux/3
  In4/1 -> Mux/4
  In6/1 -> Mux/6
  Mux/1 -> Out1/1
  Mux1/1 -> Out2/1
  In7/1 -> Mux1/1
  In8/1 -> Mux1/2
  In9/1 -> Mux1/3
  In10/1 -> Mux1/4
  In11/1 -> Mux1/5
  In12/1 -> Mux1/6

== system PvtSubSys_VSM_ALL/Subsystem/StateManage/LSS/TargetLineSelect/LCKLineS9 ==
  In1 : Inport
  In2 : Inport  Port=2
  In3 : Inport  Port=3
  In4 : Inport  Port=4
  In5 : Inport  Port=5
  In6 : Inport  Port=6
  In7 : Inport  Port=7
  Action Port : ActionPort
  Add : Sum  Inputs=+-
  Mux : Mux  Inputs=6
  Out1 : Outport
  wires:
  In5/1 -> Add/1
  In7/1 -> Add/2
  Add/1 -> Mux/5
  In3/1 -> Mux/3
  In2/1 -> Mux/2
  In4/1 -> Mux/4
  In1/1 -> Mux/1
  In6/1 -> Mux/6
  Mux/1 -> Out1/1
